simulink model "sw_angle_optimizer_pulse_generator"  (R2023b)
settings: Solver=ode23t  StartTime=0.0  StopTime=0.1  MaxStep=1e-6  RelTol=1e-3
settings Model: Creator=ixale  LastModifiedBy=ixale

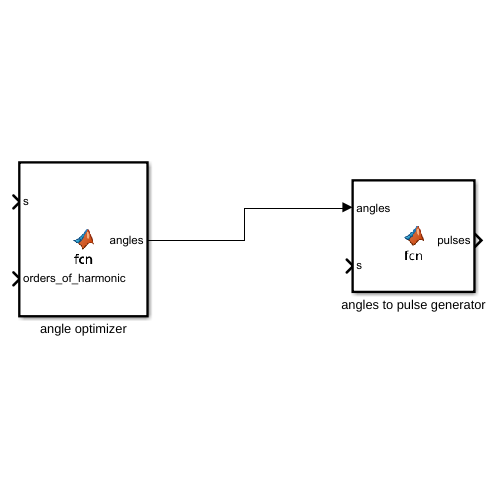
[thumbnail: Simulink's stored preview of the top-level diagram]
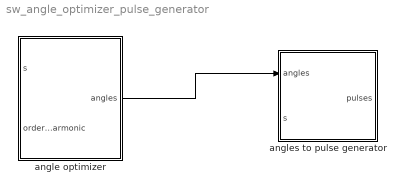
== system sw_angle_optimizer_pulse_generator ==
  angle optimizer : MATLAB Function  TreatAsAtomicUnit=on
  angles to pulse generator : MATLAB Function  TreatAsAtomicUnit=on
  wires:
  angle optimizer/1(angles) -> angles to pulse generator/1(angles)

== matlab function sw_angle_optimizer_pulse_generator/angle optimizer ==
  data: angles output; s input; orders_of_harmonic input
function angles  = fcn(s, orders_of_harmonic)

no_of_angles = s - 1;

angles = [];

function [thd] = find_thd(angles)
    thd = 0;
    i = 1;
    for angle = angles
        
        thd -= (cos(angle)* (-1).^i);
        i = i+1;
    end
end
    
for i = 1:1:no_of_angles
    angles(1) = 1;

for order = orders_of_harmonic

    for j = 1: 1 : no_of_angles
        while

== matlab function sw_angle_optimizer_pulse_generator/angles to pulse generator ==
  data: angles input; pulses output; s input
function pulses  = fcn(angles, s)

pulses = [1,0,1];
